simulink model "variable_delay"  (R2017b)
settings: Solver=VariableStepAuto  StartTime=0.0  StopTime=10.0  RelTol=1e-3  EnableMultiTasking=on
libraries: dspsigops x4
settings Model: Creator=qlong1505  LastModifiedBy=e25756
settings DataIOCC: LimitDataPoints=on
settings OptimizationCC: LifeSpan=inf
settings DebuggingCC: AllowSymbolicDim=off  SFUnexpectedBacktrackingDiag=warning  SFNoUnconditionalDefaultTransitionDiag=warning  SFExecutionAtInitializationDiag=none
settings ModelReferenceCC: PropagateSignalLabelsOutOfModel=off
settings CodeAppCC: StateflowObjectComments=on
settings GRTTargetCC: TargetLangStandard=C89/C90 (ANSI)
settings ConfigComp: CovMetricSettings=dw  CovHtmlReporting=on  CovSaveCumulativeToWorkspaceVar=on  CovSaveSingleToWorkspaceVar=on  CovExternalEMLEnable=off

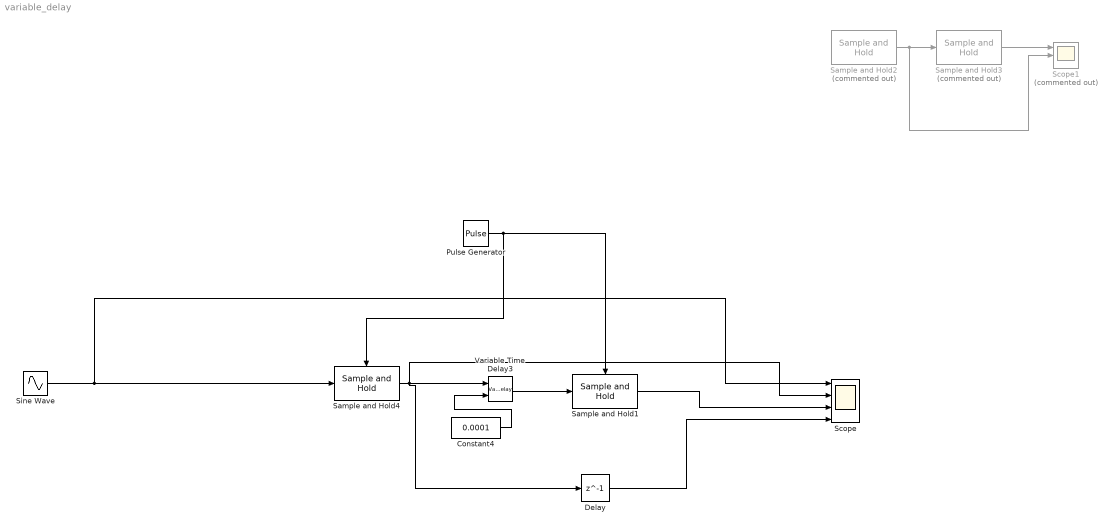
== system variable_delay ==
  Constant4 : Constant  Value=0.0001  SampleTime=0.01
  Delay : Delay  DelayLength=1  SampleTime=0.5
  Pulse Generator : DiscretePulseGenerator  PulseType=Time based  Period=0.5  PulseWidth=50
  Sample and Hold1 : dspsigops/Sample and Hold  trig=Rising edge  initCond=0  latchinput=on
  Sample and Hold2 : dspsigops/Sample and Hold  Commented=on  trig=Rising edge  initCond=0  latchinput=on
  Sample and Hold3 : dspsigops/Sample and Hold  Commented=on  trig=Rising edge  initCond=0  latchinput=on
  Sample and Hold4 : dspsigops/Sample and Hold  trig=Rising edge  initCond=0  latchinput=on
  Scope : Scope  NumInputPorts=4
  Scope1 : Scope  Commented=on  NumInputPorts=3
  Sine Wave : Sin  Frequency=2*pi/8  SampleTime=0
  Variable Time Delay3 : VariableTransportDelay  MaximumDelay=10
  wires:
  Constant4/1 -> Variable Time Delay3/2
  Sample and Hold4/1 -> Scope/2, Delay/1, Variable Time Delay3/1
  Sine Wave/1 -> Scope/1, Sample and Hold4/1
  Pulse Generator/1 -> Sample and Hold4/Trigger, Sample and Hold1/Trigger
  Variable Time Delay3/1 -> Sample and Hold1/1
  Sample and Hold1/1 -> Scope/3
  Sample and Hold2/1 -> Scope1/2, Sample and Hold3/1
  Sample and Hold3/1 -> Scope1/1
  Delay/1 -> Scope/4
